simulink library "Sys_CMD"  (R2015a)
settings: Solver=ode45  StartTime=0.0  StopTime=10.0  RelTol=1e-3
settings Model: CovModelRefEnable=off  Creator=ericli  LastModifiedBy=ericli
settings DataIOCC: SaveFormat=Dataset
settings HardwareCC: ProdBitPerPointer=64  ProdLargestAtomicFloat=Float  ProdIntDivRoundTo=Zero  ProdEndianess=LittleEndian  ProdHWDeviceType=Specified
settings GRTTargetCC: GeneratePreprocessorConditionals=Use local settings

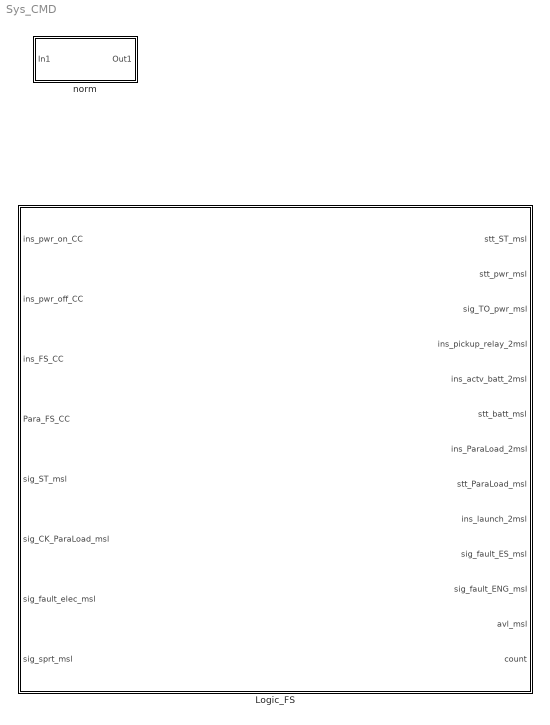
== system Sys_CMD ==
  Logic_FS : Stateflow chart  TreatAsAtomicUnit=on
  norm : Subsystem  TreatAsAtomicUnit=on
      mask DialogControl DescTextVar Prompt: 二范数%<MaskDescription>

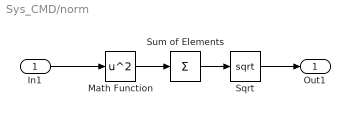
== system Sys_CMD/norm ==
  In1 : Inport
  Math Function : Math  Operator=square  SaturateOnIntegerOverflow=on
  Sqrt : Sqrt  SaturateOnIntegerOverflow=on
  Sum of Elements : Sum  Inputs=+
  Out1 : Outport
  wires:
  In1/1 -> Math Function/1
  Math Function/1 -> Sum of Elements/1
  Sum of Elements/1 -> Sqrt/1
  Sqrt/1 -> Out1/1

== stateflow chart Sys_CMD/Logic_FS ==
  state FS [group]
    state relay
      en,du: ins_pickup_relay_2msl = true;
    state batt_actv
      en,du: ins_actv_batt_2msl = true;
    state para_load1
      en,du: ins_ParaLoad_2msl = true;
    state para_check
      en,du: ins_ParaLoad_2msl = true;
    state para_load2
      en,du: ins_ParaLoad_2msl = true;
    state launch
      en: stt_ParaLoad_msl = true;
      en,du:
      stt_ParaLoad_msl = true;
      ins_launch_2msl = true;
    state timer_seprate
      en:
      avl_msl = false;
      count = 0;
      du:
      count = count+1;
    relay -> batt_actv : after(2,sec)
    batt_actv -> para_load1 : after(2,sec){stt_batt_msl = true}
    para_load1 -> para_check : after(2,sec)
    para_load2 -> (junction 63) : after(2,sec)
    (junction 57) -> para_load2 [order 2]
    para_check -> (junction 57) : after(2,sec)
    (junction 57) -> launch [order 1] : [sig_CK_ParaLoad_msl]
    (junction 63) -> (junction 70) [order 2]
    (junction 63) -> launch [order 1] : [sig_CK_ParaLoad_msl]
    (junction 68) -> (junction 70) [order 2] : {
        | sig_fault_ENG_msl = true;
        | }
    launch -> (junction 68) : after(0.5,sec)
    (junction 68) -> timer_seprate [order 1] : [sig_sprt_msl]
  state during
    en: stt_ST_msl = true;
  state prepare
  state pwron
    en: stt_pwr_msl = true;
  state pwroff
    en: stt_pwr_msl = false;
  state unavailable
    en: avl_msl = false;
  note: 图中自检结果的条件为暂定：
      | sig_ST_msl，自检结果应该有三种情况，未收到自检结果，收到的自检结果正常，收到的自检结果不正常
  (default) -> prepare : {
      | avl_msl = true;
      | }
  during -> relay [order 1] : [ins_FS_CC]
  pwron -> (junction 76) : after(0.5,sec)
  (junction 76) -> during [order 1] : [sig_ST_msl]
  prepare -> pwron : [ins_pwr_on_CC]
  (junction 76) -> pwroff [order 2] : {
      | stt_ST_msl = false;
      | }
  during -> (junction 34) [order 2] : after(30*60,sec){sig_TO_pwr_msl = true}
  (junction 79) -> prepare [order 2]
  (junction 34) -> pwroff : [ins_pwr_off_CC]
  (junction 70) -> pwroff : {
      | sig_fault_ES_msl = true;
      | }
  pwroff -> (junction 79) : after(0.5,sec)
  (junction 79) -> unavailable [order 1] : [sig_fault_ES_msl || sig_fault_ENG_msl]
  data: stt_ST_msl output boolean; stt_pwr_msl output boolean; sig_TO_pwr_msl output boolean; ins_pickup_relay_2msl output boolean; ins_actv_batt_2msl output boolean; stt_batt_msl output boolean; ins_ParaLoad_2msl output boolean; stt_ParaLoad_msl output boolean; ins_launch_2msl output boolean; sig_fault_ES_msl output boolean; ins_pwr_on_CC input; ins_pwr_off_CC input; ins_FS_CC input; Para_FS_CC input; sig_ST_msl input; sig_CK_ParaLoad_msl input; sig_fault_elec_msl input; sig_fault_ENG_msl output boolean; sig_sprt_msl input; avl_msl output boolean; count output double
